simulink model "fangzheng_run_2024a"  (R2024a)
settings: Solver=ode5  StartTime=0.0  StopTime=600  FixedStep=0.05  RelTol=1e-3
values from neighbouring files (symbols this model uses):
  Ini_Omega = 1.59    [fangzheng.m]    (also in setup_sim.m)
  J_total = Jr + (ng^2) * Jg    (= 464744.67254)    [fangzheng.m]    (also in setup_sim.m = 504744.67254)
  R = 20    [fangzheng.m]    (also in setup_sim.m)
  rho = 1.225    [fangzheng.m]    (also in setup_sim.m)
  use_raw_flag = false    [fangzheng.m]
settings Model: Creator=ADMIN  LastModifiedBy=elaina
settings DataIOCC: ReturnWorkspaceOutputs=off

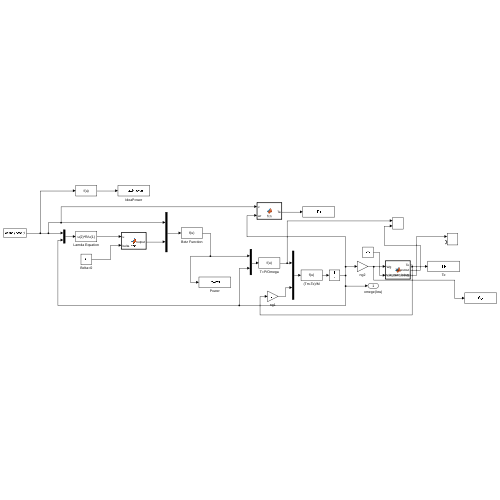
[thumbnail: Simulink's stored preview of the top-level diagram]
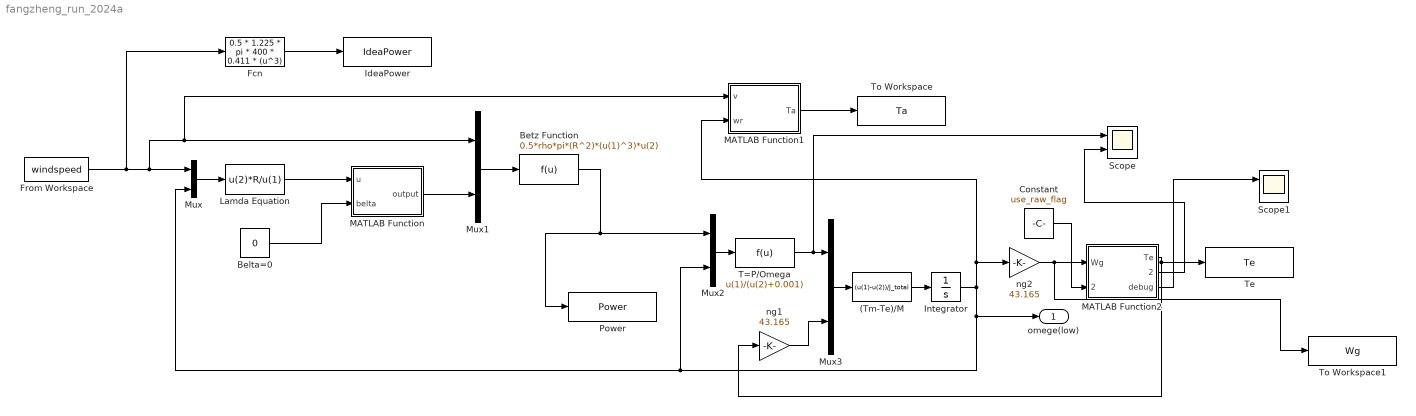
== system fangzheng_run_2024a ==
  (Tm-Te)/M : Fcn  Expr=(u(1)-u(2))/J_total
  Belta=0 : Constant  Value=0
  Betz Function : Fcn  Expr=0.5*rho*pi*(R^2)*(u(1)^3)*u(2)
  Constant : Constant  Value=use_raw_flag
  Fcn : Fcn  Expr=0.5 * 1.225 * pi * 400 * 0.411 * (u^3)
  From Workspace : FromWorkspace  VariableName=windspeed
  IdeaPower : ToWorkspace  VariableName=IdeaPower  SaveFormat=Timeseries  SampleTime=-1
  Integrator : Integrator  InitialCondition=Ini_Omega
  Lamda Equation : Fcn  Expr=u(2)*R/u(1)
  MATLAB Function : MATLAB Function  TreatAsAtomicUnit=on
  MATLAB Function1 : MATLAB Function  TreatAsAtomicUnit=on
  MATLAB Function2 : MATLAB Function  TreatAsAtomicUnit=on  SystemSampleTime=0.05
  Mux{,1..3} (4 alike) : Mux  Inputs=2
  Power : ToWorkspace  VariableName=Power  SaveFormat=Timeseries  SampleTime=-1
  Scope : Scope  NumInputPorts=2
  Scope1 : Scope  NumInputPorts=2
  T=P/Omega : Fcn  Expr=u(1)/(u(2)+0.001)
  Te : ToWorkspace  VariableName=Te  SampleTime=-1
  To Workspace : ToWorkspace  VariableName=Ta  SaveFormat=Timeseries  SampleTime=-1
  To Workspace1 : ToWorkspace  VariableName=Wg  SaveFormat=Timeseries  SampleTime=-1
  ng1 : Gain  Gain=43.165
  ng2 : Gain  Gain=43.165
  omege(low) : Outport
  wires:
  From Workspace/1 -> Fcn/1, MATLAB Function1/1(v), Mux1/1, Mux/1
  Belta=0/1 -> MATLAB Function/2(belta)
  Mux/1 -> Lamda Equation/1
  Lamda Equation/1 -> MATLAB Function/1(u)
  MATLAB Function/1(output) -> Mux1/2
  Mux1/1 -> Betz Function/1
  Betz Function/1 -> Power/1, Mux2/1
  Mux2/1 -> T=P/Omega/1
  Mux3/1 -> (Tm-Te)/M/1
  (Tm-Te)/M/1 -> Integrator/1
  T=P/Omega/1 -> Scope/1, Mux3/1
  ng2/1 -> To Workspace1/1, MATLAB Function2/1(Wg)
  MATLAB Function2/1(Te) -> ng1/1, Te/1
  Fcn/1 -> IdeaPower/1
  Integrator/1 -> MATLAB Function1/2(wr), ng2/1, Mux2/2, Mux/2, omege(low)/1
  MATLAB Function1/1(Ta) -> To Workspace/1
  ng1/1 -> Mux3/2
  MATLAB Function2/2(Ta_estout) -> Scope/2
  MATLAB Function2/3(debug) -> Scope1/1
  Constant/1 -> MATLAB Function2/2(use_raw)

== matlab function fangzheng_run_2024a/MATLAB Function1 ==
  data: v input; Ta output; wr input
function Ta = fcn(v, wr)
% 这是一个计算风机气动转矩的模块
% 输入 v : 实时风速 (m/s)
% 输入 wr: 低速轴风轮转速 (rad/s)
% 输出 Ta: 气动转矩 (Nm)

% 1. 定义 600kW 风机的固有参数
R = 20;           % 风轮半径 (m)
rho = 1.225;      % 空气密度 (kg/m^3)
beta = 0;         % 桨距角 (MPPT阶段通常恒为0度)

% 2. 容错处理：防止仿真初期转速或风速为0导致除以零报错
if v < 0.1
    v = 0.1;
end
if wr < 0.1
    wr = 0.1;
end

% 3. 计算叶尖速比 Lambda
lambda = (wr * R) / v;

% 4. 计算风能利用系数 Cp
% （这里使用的是风电领域最经典通用的 Cp 解析函数，你也可以替换成你课件上特定的公式）
lambda_i = 1 / (1 / (lambda + 0.08 * beta) - 0.035 / (beta^3 + 1));
Cp = 0.5176 * (116 / lambda_i - 0.4 * beta - 5) * exp(-21 / lambda_i) + 0.0068 * lambda;

% 限制 Cp 的下限，防止出现发电机倒拖风轮的负功率现象
if Cp < 0
    Cp = 0;
end

% 5. 计算气动功率 Pa 和 气动转矩 Ta
Pa = 0.5 * rho * pi * R^2 * v^3 * Cp;
Ta = Pa / wr;

end

== matlab function fangzheng_run_2024a/MATLAB Function ==
  data: u input; output output; belta input
function output = fcn(u, belta)
    % u 对应叶尖速比 lambda，belta 对应桨距角 beta
    
    % 直接计算 1/A 的整体值，命名为 invA
    invA = 1 / (u + 0.08 * belta) - 0.035;
    
    % 注意：指数必须使用 exp() 函数
    C_p = 0.5 * (116 * invA - 0.4 * belta - 5) * exp(-21 * invA);
    
    % 防止物理上不可能的负风能捕获
    if C_p < 0
        C_p = 0;
    end
    
    output = C_p;
end

== matlab function fangzheng_run_2024a/MATLAB Function2 ==
  data: Wg input; Te output; Ta_estout output; debug output; use_raw input
function [Te, Ta_estout,debug] = fcn_instant_custom(Wg,use_raw)
    
    % 1. 预定义/初始化输出变量 (这一步是关键)
    % 假设你的输出都是标量 double，如果不是，请按实际维度修改
    Te = 0.0; 
    Ta_estout = 0.0;
    debug = 0.0; 
    coder.extrinsic('mppt_raw');
    coder.extrinsic('mppt_enhance');
    if use_raw
        
        Te=mppt_raw(Wg);
        Ta_estout = 0.0; % 或者给一个特定的默认值
        debug = 0.0;
    else
        
         % 2. 声明外部函数
       

        % 3. 调用外部函数
        [Te, Ta_estout, debug] = mppt_enhance(Wg);
    end
end
